simulink model "canard"  (R2023b)
settings: Solver=VariableStepAuto  StartTime=0.0  StopTime=60  RelTol=1e-3
values from neighbouring files (symbols this model uses):
  L_p = -0.1    [params.m]
  p_c = 0    [params.m]
  q_c = 0    [params.m]
  r_c = 0    [params.m]
  t_act = 10.0    (= 10)    [params.m]
libraries: simulink x2, slpidlib x1
settings Model: Creator=joedo  LastModifiedBy=joedo

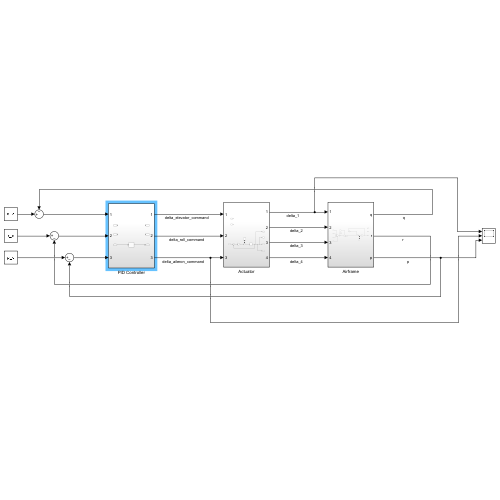
[thumbnail: Simulink's stored preview of the top-level diagram]
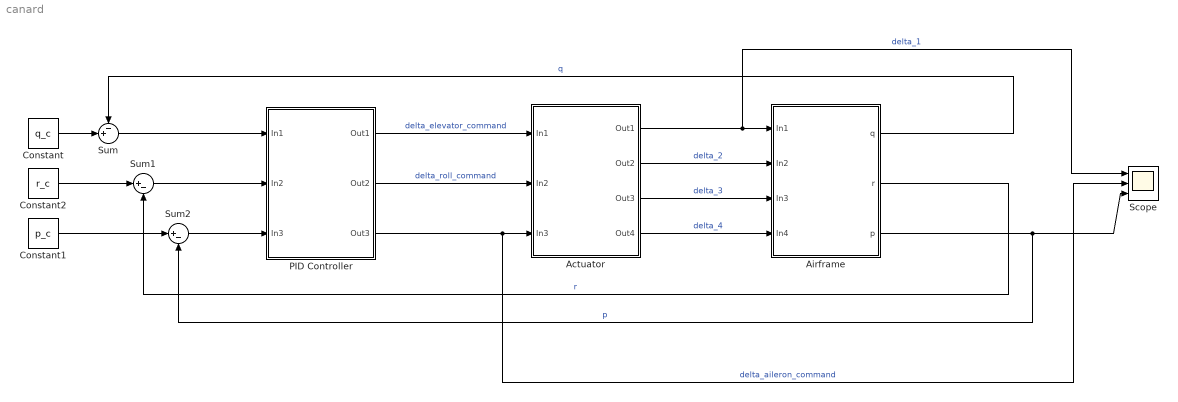
== system canard ==
  Actuator : Subsystem
  Airframe : Subsystem
  Constant : Constant  Value=q_c
  Constant1 : Constant  Value=p_c
  Constant2 : Constant  Value=r_c
  PID Controller : Subsystem
  Scope : Scope  NumInputPorts=3
  Sum : Sum  Inputs=-+|
  Sum1 : Sum  Inputs=|+-
  Sum2 : Sum  Inputs=|+-
  wires:
  Constant2/1 -> Sum1/1
  Constant/1 -> Sum/2
  Constant1/1 -> Sum2/1
  Sum/1 -> PID Controller/1(In1)
  Sum1/1 -> PID Controller/2(In2)
  Sum2/1 -> PID Controller/3(In3)
  PID Controller/1(Out1) -> Actuator/1(In1)  "delta_elevator_command"
  PID Controller/2(Out2) -> Actuator/2(In2)  "delta_roll_command"
  PID Controller/3(Out3) -> Scope/2, Actuator/3(In3)  "delta_aileron_command"
  Actuator/4(Out4) -> Airframe/4(In4)  "delta_4"
  Actuator/3(Out3) -> Airframe/3(In3)  "delta_3"
  Actuator/2(Out2) -> Airframe/2(In2)  "delta_2"
  Actuator/1(Out1) -> Scope/1, Airframe/1(In1)  "delta_1"
  Airframe/1(q) -> Sum/1  "q"
  Airframe/2(r) -> Sum1/2  "r"
  Airframe/3(p) -> Scope/3, Sum2/2  "p"

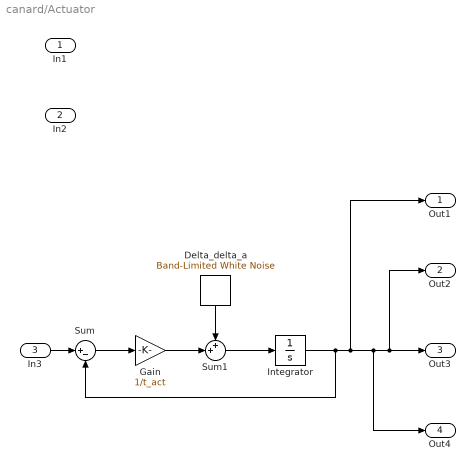
== system canard/Actuator ==
  In1 : Inport
  In2 : Inport  Port=2
  In3 : Inport  Port=3
  Delta_delta_a : simulink/Sources/Band-Limited White Noise  Cov=[0.01]  Ts=0.1  seed=[23341]
  Gain : Gain  Gain=1/t_act
  Integrator : Integrator
  Sum : Sum  Inputs=|+-
  Sum1 : Sum  Inputs=++|
  Out1 : Outport
  Out2 : Outport  Port=2
  Out3 : Outport  Port=3
  Out4 : Outport  Port=4
  wires:
  In3/1 -> Sum/1
  Integrator/1 -> Sum/2, Out1/1, Out4/1, Out2/1, Out3/1
  Gain/1 -> Sum1/2
  Sum/1 -> Gain/1
  Sum1/1 -> Integrator/1
  Delta_delta_a/1 -> Sum1/1

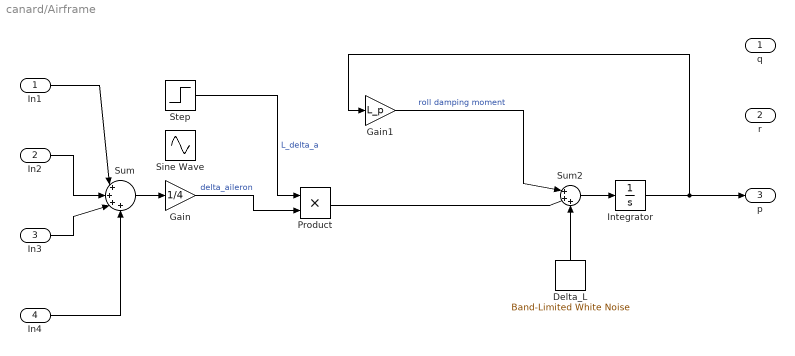
== system canard/Airframe ==
  In1 : Inport
  In2 : Inport  Port=2
  In3 : Inport  Port=3
  In4 : Inport  Port=4
  Delta_L : simulink/Sources/Band-Limited White Noise  Cov=[0.01]  Ts=0.1  seed=[23341]
  Gain : Gain  Gain=1/4
  Gain1 : Gain  Gain=L_p
  Integrator : Integrator  InitialCondition=5
  Product : Product
  Sine Wave : Sin  SampleTime=0
  Step : Step  SampleTime=0
  Sum : Sum  Inputs=|++++
  Sum2 : Sum  Inputs=|+++
  q : Outport
  r : Outport  Port=2
  p : Outport  Port=3
  wires:
  Sum/1 -> Gain/1
  In1/1 -> Sum/1
  In2/1 -> Sum/2
  In3/1 -> Sum/3
  In4/1 -> Sum/4
  Gain/1 -> Product/2  "delta_aileron"
  Integrator/1 -> Gain1/1, p/1
  Step/1 -> Product/1  "L_delta_a"
  Sum2/1 -> Integrator/1
  Delta_L/1 -> Sum2/3
  Product/1 -> Sum2/2
  Gain1/1 -> Sum2/1  "roll damping moment"

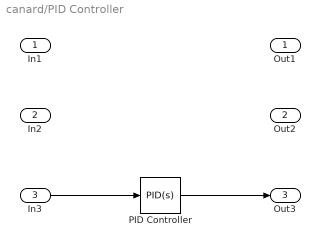
== system canard/PID Controller ==
  In1 : Inport
  In2 : Inport  Port=2
  In3 : Inport  Port=3
  PID Controller : slpidlib/PID Controller  Controller=PID  Form=Parallel  TimeDomain=Continuous-time  UseExternalTs=off  SampleTime=-1  IntegratorMethod=Forward Euler  FilterMethod=Forward Euler  ControllerParametersSource=internal  P=1  I=0.05  UseKiTs=off  D=0.2  N=100  UseFilter=on  TunerSelectOption=Transfer Function Based (PID Tuner App)  InitialConditionSource=internal  InitialConditionForIntegrator=0  InitialConditionForFilter=0  DifferentiatorICPrevScaledInput=0  ExternalReset=none  TrackingMode=off  Kt=1  LimitOutput=on  SatLimitsSource=internal  UpperSaturationLimit=5  LowerSaturationLimit=-5  LinearizeAsGain=on  AntiWindupMode=none  Kb=1  LimitIntegrator=off  UpperIntegratorSaturationLimit=inf  LowerIntegratorSaturationLimit=-inf  POutMin=[]  POutMax=[]  IOutMin=[]  IOutMax=[]  DOutMin=[]  DOutMax=[]  NOutMin=[]  NOutMax=[]  SumOutMin=[]  SumOutMax=[]  SaturationOutMin=[]  SaturationOutMax=[]  PParamMin=[]  PParamMax=[]  IParamMin=[]  IParamMax=[]  DParamMin=[]  DParamMax=[]  NParamMin=[]  NParamMax=[]  KbParamMin=[]  KbParamMax=[]  KtParamMin=[]  KtParamMax=[]  KbOutMin=[]  KbOutMax=[]  KtOutMin=[]  KtOutMax=[]  IntegratorOutMin=[]  IntegratorOutMax=[]  FilterOutMin=[]  FilterOutMax=[]  SumI1OutMin=[]  SumI1OutMax=[]  SumI2OutMin=[]  SumI2OutMax=[]  SumI3OutMin=[]  SumI3OutMax=[]  SumI4OutMin=[]  SumI4OutMax=[]  SumDOutMin=[]  SumDOutMax=[]  DifferentiatorOutMin=[]  DifferentiatorOutMax=[]  FilterDiffOutCoefMin=[]  FilterDiffOutCoefMax=[]  ReciprocalOutMin=[]  ReciprocalOutMax=[]  SumDenOutMin=[]  SumDenOutMax=[]  SumNumOutMin=[]  SumNumOutMax=[]  DivideOutMin=[]  DivideOutMax=[]  UdiffTsProdOutMin=[]  UdiffTsProdOutMax=[]  NTsProdOutMin=[]  NTsProdOutMax=[]  UintegralTsProdOutMin=[]  UintegralTsProdOutMax=[]  UngainTsProdOutMin=[]  UngainTsProdOutMax=[]  ClampingZeroOutDataTypeStr=Inherit: Inherit via back propagation  ClampingZeroOutMin=[]  ClampingZeroOutMax=[]  FilterDenConstantOutDataTypeStr=Inherit: Inherit via back propagation  FilterDenConstantOutMin=[]  FilterDenConstantOutMax=[]  PCopyOutDataTypeStr=Inherit: Inherit via back propagation  PCopyOutMin=[]  PCopyOutMax=[]  NCopyOutDataTypeStr=Inherit: Inherit via back propagation  NCopyOutMin=[]  NCopyOutMax=[]  IntegratorContinuousStateAttributes=''  IntegratorStateMustResolveToSignalObject=off  IntegratorRTWStateStorageClass=Auto  FilterContinuousStateAttributes=''  FilterStateMustResolveToSignalObject=off  FilterRTWStateStorageClass=Auto  ParallelPVariant=InternalParameters  IdealPVariant=Disabled  IVariant=InternalParameters  DVariant=InternalParameters  IntegratorVariant=Continuous  SatVariant=Enabled  AWVariant=Passthrough  PCopyVariant=Disabled  TRVariant=Disabled  FdbkBlocksVariant=Forward  IdealPFdbkVariant=Disabled  SatFdbkVariant=Disabled  DerivativeFilterVariant=ContFilter  NVariant=InternalParameters  NCopyVariant=Disabled  FilterICVariant=InternalICsFilter  IntegratorICVariant=InternalICs  ExternalResetVariant=Disabled  TRSumVariant=Passthrough  SumFdbkVariant=Disabled  SumVariant=Sum_PID  TsampFilterVariant=InternalTs  TsampNgainVariant=Passthrough  TsampIntegralVariant=Disabled_SignalSpec  ExternalSaturationOutDataTypeStr=Inherit: Same as second input
  Out1 : Outport
  Out2 : Outport  Port=2
  Out3 : Outport  Port=3
  wires:
  In3/1 -> PID Controller/1
  PID Controller/1 -> Out3/1
